simulink model "Auto_microgrid_forecasting_020822"  (R2020a)
settings: Solver=VariableStepAuto  StartTime=0.0  StopTime=50  MaxStep=1e-4  RelTol=1e-3
PreLoadFcn:
  | %run('FC_microgrid_param.m')
  | %load('gen_grid_init.mat')
InitFcn:
  | %load myisoModel_init;
  | run('FC_microgrid_param.m')
  | tic
  | run('CARTinitFcn.m')
  | %caseNo = 2;
  | 
  | %if (caseNo == 1)
  | %set_param(['Isolated_grid_paper_model_022521/SignalGen'], 'ActiveScenario', 'PStep222kW');
  | %else
  | %set_param(['Isolated_grid_paper_model_022521/SignalGen'], 'ActiveScenario', 'QStep222kVAr');
  | 
  | %end;
StopFcn:
  | toc
undefined symbols (not defined in the file or in its folder): breakpoints1, breakpoints2, cc_kp, cp_table_data, ctrl, D1, Delta, DiscIntNeverNeededParam, DT, FC_BESS, FC_PV_FirstSolar, find_system, Fnom, gcbh, libFC_BESS, libFC_PV, LowerLimit, magnitude, oversize, pll_ki, pll_kp, pq_ts, SOC_target, sps_rtmsupport, timer, Ts, ts, Ts_APC, Ts_Control, Ts_Power, UpperLimit
libraries: powerlib x151, simulink x100, powerlib_extras x100, powerlib_meascontrol x91, eePowerMeasurement x26, pi_ctrl x16, simulink_extras x12, sps_avr x7, eeGeneralControl x5, spsDieselMotorModel x3, libFSArray x2, SignalEditorBlockLib x2
(part 2 of 14)

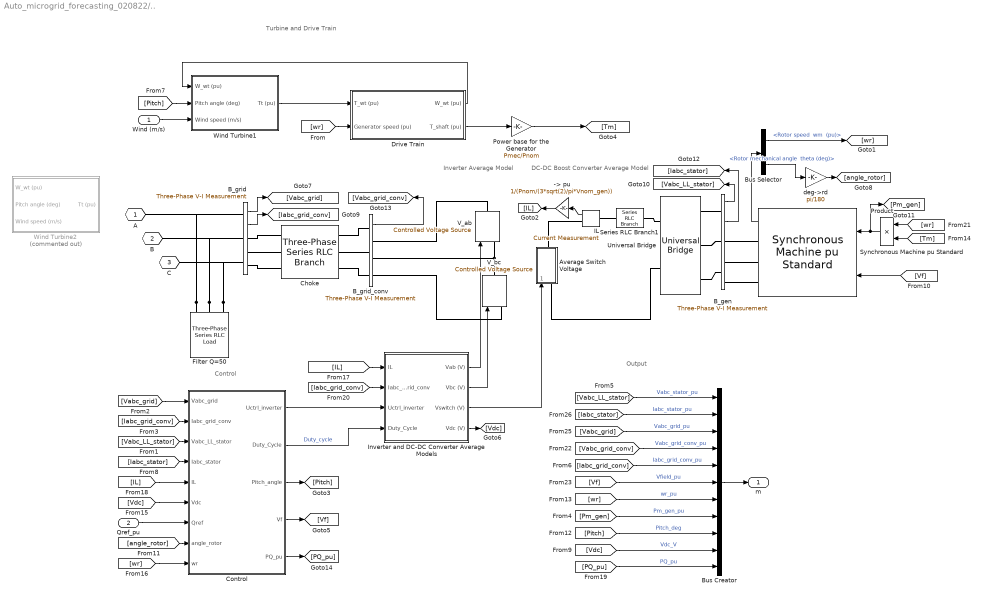
== system Auto_microgrid_forecasting_020822/.. ==
  note: DC-DC Boost Converter
      | Average Model
  note: Inverter
      | Average Model
  note: Output
  note: Control
  note: Turbine and Drive Train
  "Wind (m/s) " : Inport
  Qref_pu : Inport  Port=2
  -> pu : Gain  Gain=1/(Pnom/(3*sqrt(2)/pi*Vnom_gen))  SaturateOnIntegerOverflow=on  OutDataTypeStr=Inherit: Same as input  ParamDataTypeStr=Inherit: Same as input
  Average Switch Voltage : Subsystem
  B_gen : powerlib/Measurements/Three-Phase V-I Measurement  VoltageMeasurement=phase-to-phase  SetLabelV=off  LabelV=Vabc  Vpu=on  VpuLL=off  CurrentMeasurement=yes  SetLabelI=off  LabelI=Iabc  Ipu=on  Pbase=Pnom  Vbase=Vnom_gen  OutputType=Complex  PhasorSimulation=off  PSBequivalent=0
      settings: SourceProductBaseCode=MT,PS
  B_grid : powerlib/Measurements/Three-Phase V-I Measurement  VoltageMeasurement=phase-to-ground  SetLabelV=off  LabelV=Vabc  Vpu=on  VpuLL=off  CurrentMeasurement=yes  SetLabelI=off  LabelI=Iabc  Ipu=on  Pbase=Pnom  Vbase=Vnom  OutputType=Complex  PhasorSimulation=off  PSBequivalent=0
      settings: SourceProductBaseCode=MT,PS
  B_grid_conv : powerlib/Measurements/Three-Phase V-I Measurement  VoltageMeasurement=phase-to-ground  SetLabelV=off  LabelV=Vabc  Vpu=on  VpuLL=off  CurrentMeasurement=no  SetLabelI=off  LabelI=Iabc  Ipu=on  Pbase=Pnom  Vbase=Vnom  OutputType=Complex  PhasorSimulation=off  PSBequivalent=0
      settings: SourceProductBaseCode=MT,PS
  Bus Creator : BusCreator  Inputs=11
  Bus Selector : BusSelector  OutputSignals="Mechanical.Rotor speed  wm  (pu),Mechanical.Rotor mechanical angle  theta (deg)"
  "Choke " : powerlib/Elements/Three-Phase Series RLC Branch  LConnTagsString=A|B|C  RConnTagsString=A|B|C  BranchType=RL  Resistance=R_RL*Vnom^2/Pnom  Inductance=L_RL*Vnom^2/Pnom/(2*pi*Fnom)  Capacitance=[]  Measurements=None
      settings: SourceProductBaseCode=MT,PS
  Control : Subsystem
  Drive Train : Subsystem  mask(Wind Turbine shaft){H_WT=H_WT, Ksh=Ksh, D_mutual=D_mutual, wbase=2*pi*Fnom/p, w_wt0=w_wt0, torque0=torque0, Ts=Ts}
      mask prompts: H_WT "Wind turbine inertia constant H (s):"; Ksh "Shaft spring constant (pu of nominal mechanical torque/rad):"; D_mutual "Shaft mutual damping (pu of nominal mechanical torque/pu dw):"; wbase "Shaft base speed (rad/s):"; w_wt0 "Turbine initial speed (pu of base speed):"; torque0 "Initial output torque (pu of nominal mechanical torque):"; Ts "Sample time (s):"
      mask help:
      | This block implements a wind turbine drive train model. All shaft parameters are referred to high-speed shaft (generator shaft).
      |
      | The first input is the wind turbine torque in per unit (pu) based on the nominal power of the turbine and the base speed of the generator. The second input is the generator speed in pu based on the base speed of the generator.
      |
      | The outputs are:
      | 1- the transmitted torque of the shaft in pu based on the nominal power of the turbine and the base speed of the generator.
      | 2- the wind turbine speed in pu of the base speed of the generator.
  Filter Q=50 : powerlib/Elements/Three-Phase Series RLC Load  LConnTagsString=A|B|C  Configuration=Y (grounded)  NominalVoltage=Vnom  Vabc=[1e3 1e3 1e3]  Vabcp=[1e3 1e3 1e3]  NominalFrequency=Fnom  UnbalancedPower=off  ActivePower=C_var_filter/Q_filter  InductivePower=0  CapacitivePower=C_var_filter  Pabc=[10e3 9e3 11e3]  QLabc=[100 90 110]  QCabc=[100 90 110]  Pabcp=[10e3 9e3 11e3]  QLabcp=[100 90 110]  QCabcp=[100 90 110]  Measurements=None  LoadType=constant Z
      settings: SourceProductBaseCode=MT,PS
  IL : powerlib/Measurements/Current Measurement  PhasorSimulation=off  OutputType=Complex  PSBequivalent=0
      settings: SourceProductBaseCode=MT,PS
  Inverter and DC-DC Converter Average Models : Subsystem
  Power base for the Generator : Gain  Gain=Pmec/Pnom  SaturateOnIntegerOverflow=on  OutDataTypeStr=Inherit: Same as input  ParamDataTypeStr=Inherit: Same as input
  Product : Product  RndMeth=Zero
  Series RLC Branch1 : powerlib/Elements/Series RLC Branch  LConnTagsString=__new0  RConnTagsString=__new0  BranchType=RL  Resistance=R_Boost  Inductance=L_Boost  SetiL0=off  InitialCurrent=0  Capacitance=1.0  Setx0=off  InitialVoltage=0  Measurements=Branch current
      settings: SourceProductBaseCode=MT,PS
  Synchronous Machine pu Standard : powerlib/Machines/Synchronous Machine pu Standard  PresetModel=No  MechanicalLoad=Mechanical power Pm  ShowDetailedParameters=on  RotorType=Salient-pole  Units=per unit standard parameters  MeasurementBus=off  NominalParameters="[ Pnom  Vnom_gen Fnom ]"  Reactances1=[ 1.81, 0.3, 0.23, 1.76, 0.65, 0.25, 0.15 ]  Reactances2="[ Xd, Xd1, Xd2, Xq,  Xq2,  Xl ]"  dAxisTimeConstants=Open-circuit  qAxisTimeConstants=Short-circuit  TimeConstants1="[ 4.4849  0.0681  0.1  ]"  TimeConstants2=[ 8.0, 0.03, 1.0, 0.07 ]  TimeConstants3="[  Tdo1  Tdo2  Tq2  ]"  TimeConstants4=[ 8.0, 0.03, 0.3371, 0.0295 ]  TimeConstants5=[ 1.01, 0.053, 0.1 ]  TimeConstants6=[ 1.3201, 0.023, 1.0, 0.07 ]  TimeConstants7="[  1.01  0.053  0.051266  ]"  TimeConstants8=[ 1.3201, 0.0231, 0.3371, 0.0295 ]  StatorResistance=Resistance  Mechanical=[ H F p]  PolePairs=1  InitialConditions=init  SetSaturation=off  Saturation=[0.6404,0.7127,0.8441,0.9214,0.9956,1.082,1.19,1.316,1.457;0.7,0.7698,0.8872,0.9466,0.9969,1.046,1.1,1.151,1.201]  LoadFlowParameters=[1,0,0,0,0]  TsPowergui=0  TsBlock=-1  IterativeModel=Trapezoidal non iterative  IterativeDiscreteModel=Trapezoidal non iterative  BusType=PV  Pref=0  Qref=0  Qmin=-inf  Qmax=inf  PLF=0  QLF=0
      settings: SourceProductBaseCode=MT,PS
  Universal Bridge : powerlib/Power Electronics/Universal Bridge  Arms=3  SnubberResistance=2*Ts_snub/(Pnom/(1000*2*pi*Fnom*Vnom_gen^2))  SnubberCapacitance=Pnom/(1000*2*pi*Fnom*Vnom_gen^2)  Device=Diodes  Ron=1e-6/Nb_wt  Lon=0  ForwardVoltages="[  0  0  ]"  ForwardVoltage=0  GTOparameters=[ 10e-6 , 20e-6 ]  IGBTparameters=[ 1e-6 , 2e-6 ]  Measurements=None  Measurements_2=None  converterType=Rectifier
      settings: SourceProductBaseCode=MT,PS
  V_ab : powerlib/Electrical Sources/Controlled Voltage Source  Initialize=on  Source_Type=AC  Amplitude=0  Phase=0  Frequency=0  Measurements=None
      settings: SourceProductBaseCode=MT,PS
  V_bc : powerlib/Electrical Sources/Controlled Voltage Source  Initialize=on  Source_Type=AC  Amplitude=0  Phase=0  Frequency=0  Measurements=None
      settings: SourceProductBaseCode=MT,PS
  Wind Turbine1 : Subsystem  mask(Wind Turbine){Prated=Pmec, c1_c8=c1_c8, K1_K2=K1_K2, wind0=wind0, Ts=Ts}
      mask prompts: Prated "Nominal mechanical output power (W):"; c1_c8 "Coefficients [c1 ... c8]"; K1_K2 "Parameters [K1 K2]"; wind0 "Initial wind speed (m/s):"; Ts "Sample time (s):"
      mask help:
      | This block implements a generic wind turbine models.
      |
      | The first input is the turbine speed in per unit of the generator base speed. For a synchronous or asynchronous generator, the base speed is the synchronous speed. For a permanent-magnet generator, the base speed is defined as the speed producing nominal voltage at  no load. The second input is the blade pitch angle in degrees. The third input is the wind speed in m/s.
      |
      | The output is the torque applied to the drive train in per unit based on the nominal power of the turbine and the base speed of the generator.
      mask init:
      | c1 = c1_c8(1);
      | c2 = c1_c8(2);
      | c3 = c1_c8(3);
      | c4 = c1_c8(4);
      | c5 = c1_c8(5);
      | c6 = c1_c8(6);
      | c7 = c1_c8(7);;
      | c8 = c1_c8(8);
      | 
      | K1=K1_K2(1);
      | K2=K1_K2(2);
      settings: OpenFcn=power_openblockproxy();
      mask Display: disp('');
  Wind Turbine2 : Subsystem  Commented=on  mask(Wind Turbine){Prated=Pmec, c1_c8=c1_c8, K1_K2=K1_K2, wind0=wind0, Ts=Ts}
      mask prompts: Prated "Nominal mechanical output power (W):"; c1_c8 "Coefficients [c1 ... c8]"; K1_K2 "Parameters [K1 K2]"; wind0 "Initial wind speed (m/s):"; Ts "Sample time (s):"
      mask help:
      | This block implements a generic wind turbine models.
      |
      | The first input is the turbine speed in per unit of the generator base speed. For a synchronous or asynchronous generator, the base speed is the synchronous speed. For a permanent-magnet generator, the base speed is defined as the speed producing nominal voltage at  no load. The second input is the blade pitch angle in degrees. The third input is the wind speed in m/s.
      |
      | The output is the torque applied to the drive train in per unit based on the nominal power of the turbine and the base speed of the generator.
      mask init:
      | c1 = c1_c8(1);
      | c2 = c1_c8(2);
      | c3 = c1_c8(3);
      | c4 = c1_c8(4);
      | c5 = c1_c8(5);
      | c6 = c1_c8(6);
      | c7 = c1_c8(7);;
      | c8 = c1_c8(8);
      | 
      | K1=K1_K2(1);
      | K2=K1_K2(2);
      settings: OpenFcn=power_openblockproxy();
      mask Display: disp('');
  deg->rd : Gain  Gain=pi/180  SaturateOnIntegerOverflow=on  OutDataTypeStr=Inherit: Same as input  ParamDataTypeStr=Inherit: Same as input
  A : PMIOPort  Tag=PMCPort  Side=Left
  B : PMIOPort  Tag=PMCPort  Port=2  Side=Left
  C : PMIOPort  Tag=PMCPort  Port=3  Side=Left
  m : Outport  VectorParamsAs1DForOutWhenUnconnected=off
  wires:
  -> pu/1 -> [IL]
  [IL] -> Control/5(IL)
  [PQ_pu] -> Bus Creator/11  "PQ_pu"
  Control/5(PQ_pu) -> [PQ_pu]
  Inverter and DC-DC Converter Average Models/2(Vbc (V)) -> V_bc/1
  Inverter and DC-DC Converter Average Models/1(Vab (V)) -> V_ab/1
  [Vf] -> Synchronous Machine pu Standard/2
  Inverter and DC-DC Converter Average Models/4(Vdc (V)) -> [Vdc]
  Control/4(Vf) -> [Vf]
  Control/3(Pitch_angle) -> [Pitch]
  Control/2(Duty_Cycle) -> Inverter and DC-DC Converter Average Models/4(Duty_Cycle)  "Duty_cycle"
  Control/1(Uctrl_inverter) -> Inverter and DC-DC Converter Average Models/3(Uctrl_inverter)
  [wr] -> Control/9(wr)
  [angle_rotor] -> Control/8(angle_rotor)
  Qref_pu/1 -> Control/7(Qref)
  [Vdc] -> Control/6(Vdc)
  [Iabc_stator] -> Control/4(Iabc_stator)
  [Vabc_LL_stator] -> Control/3(Vabc_LL_stator)
  [Iabc_grid_conv] -> Control/2(Iabc_grid_conv)
  [Vabc_grid] -> Control/1(Vabc_grid)
  B_gen/2 -> [Iabc_stator]
  B_gen/1 -> [Vabc_LL_stator]
  B_grid/2 -> [Iabc_grid_conv]
  B_grid/1 -> [Vabc_grid]
  [IL] -> Inverter and DC-DC Converter Average Models/1(IL)
  IL/1 -> -> pu/1
  Inverter and DC-DC Converter Average Models/3(Vswitch (V)) -> Average Switch Voltage/1(Vswitch)
  [Iabc_grid_conv] -> Inverter and DC-DC Converter Average Models/2(Iabc_grid_conv)
  Product/1 -> [Pm_gen], Synchronous Machine pu Standard/1
  [Tm] -> Product/2
  [Vdc] -> Bus Creator/10  "Vdc_V"
  [Pitch] -> Bus Creator/9  "Pitch_deg"
  [Pm_gen] -> Bus Creator/8  "Pm_gen_pu"
  [wr] -> Bus Creator/7  "wr_pu"
  [Vf] -> Bus Creator/6  "Vfield_pu"
  [Iabc_grid_conv] -> Bus Creator/5  "Iabc_grid_conv_pu"
  [Vabc_grid_conv] -> Bus Creator/4  "Vabc_grid_conv_pu"
  Bus Creator/1 -> m/1
  [Vabc_grid] -> Bus Creator/3  "Vabc_grid_pu"
  [Iabc_stator] -> Bus Creator/2  "Iabc_stator_pu"
  [Vabc_LL_stator] -> Bus Creator/1  "Vabc_stator_pu"
  B_grid_conv/1 -> [Vabc_grid_conv]
  Synchronous Machine pu Standard/1 -> Bus Selector/1
  [wr] -> Product/1
  Bus Selector/1 -> [wr]  "<Rotor speed  wm  (pu)>"
  deg->rd/1 -> [angle_rotor]
  Bus Selector/2 -> deg->rd/1  "<Rotor mechanical angle  theta (deg)>"
  [Pitch] -> Wind Turbine1/2(Pitch angle (deg))
  Drive Train/1(W_wt (pu)) -> Wind Turbine1/1(W_wt (pu))
  "Wind (m/s) "/1 -> Wind Turbine1/3(Wind speed (m/s))
  Power base for the Generator/1 -> [Tm]
  Drive Train/2(T_shaft (pu)) -> Power base for the Generator/1
  [wr] -> Drive Train/2(Generator speed (pu))
  Wind Turbine1/1(Tt (pu)) -> Drive Train/1(T_wt (pu))
  connections:
  Average Switch Voltage/RConn1 -- IL/RConn1
  Series RLC Branch1/RConn1 -- IL/LConn1
  Universal Bridge/LConn3 -- B_gen/LConn3
  Universal Bridge/LConn2 -- B_gen/LConn2
  Universal Bridge/LConn1 -- B_gen/LConn1
  B_grid_conv/RConn2 -- V_ab/LConn1 -- V_bc/RConn1
  B_grid_conv/RConn3 -- V_bc/LConn1
  V_ab/RConn1 -- B_grid_conv/RConn1
  Average Switch Voltage/LConn1 -- Universal Bridge/RConn2
  Series RLC Branch1/LConn1 -- Universal Bridge/RConn1
  "Choke "/RConn3 -- B_grid_conv/LConn3
  "Choke "/RConn2 -- B_grid_conv/LConn2
  "Choke "/RConn1 -- B_grid_conv/LConn1
  Filter Q=50/LConn3 -- B_grid/LConn3 -- C/RConn1
  Filter Q=50/LConn2 -- B_grid/LConn2 -- B/RConn1
  Filter Q=50/LConn1 -- A/RConn1 -- B_grid/LConn1
  B_grid/RConn3 -- "Choke "/LConn3
  B_grid/RConn2 -- "Choke "/LConn2
  B_grid/RConn1 -- "Choke "/LConn1
  B_gen/RConn3 -- Synchronous Machine pu Standard/RConn3
  B_gen/RConn2 -- Synchronous Machine pu Standard/RConn2
  B_gen/RConn1 -- Synchronous Machine pu Standard/RConn1

== system Auto_microgrid_forecasting_020822/Control1 ==
  Bus Creator : BusCreator  Inputs=6
  Bus Selector : BusSelector  OutputSignals=PV PQ cmd,f setpoint,V setpoint,PV switch,PV_mode
  Constant2 : Constant  Commented=on
  Constant3 : Constant  Commented=on
  Demux1 : Demux  Outputs=2
  Step2 : Step  Before=1  After=0
  Out1 : Outport
  wires:
  Bus Selector/3 -> Bus Creator/4  "<V setpoint>"
  Bus Creator/1 -> Out1/1
  Bus Selector/2 -> Bus Creator/3  "<f setpoint>"
  Bus Selector/5 -> Bus Creator/5  "<PV_mode>"
  Demux1/2 -> Bus Creator/2  "q_ref"
  Demux1/1 -> Bus Creator/1  "p_ref"
  Bus Selector/4 -> Bus Creator/6  "<PV switch>"
  [MGCC_cmd] -> Bus Selector/1
  Bus Selector/1 -> Demux1/1  "<PV PQ cmd>"
  Constant3/1 -> ?  "V setpoint"
  Constant2/1 -> ?  "f setpoint"

== system Auto_microgrid_forecasting_020822/Control3 ==
  Bus Creator : BusCreator  Inputs=5
  Constant1 : Constant  SampleTime=-1
  Constant2 : Constant  SampleTime=-1
  Constant3 : Constant  Value=-1  SampleTime=-1
  Constant5 : Constant  Value=0  SampleTime=-1
  Step1 : Step  Time=1000
  Control : Outport
  wires:
  Constant3/1 -> Bus Creator/1  "p_ref"
  Constant5/1 -> Bus Creator/2  "q_ref"
  Step1/1 -> Bus Creator/5  "GF_mode"
  Constant1/1 -> Bus Creator/3  "f_ref"
  Bus Creator/1 -> Control/1
  Constant2/1 -> Bus Creator/4  "v_ref"

== system Auto_microgrid_forecasting_020822/Defferable Load (0-446.25 kW) ==
  Control : Inport
  Demux : Demux  Outputs=8
      settings: DisplayOption=none
  Resistive Loads : Subsystem
  Switches : Subsystem
  A : PMIOPort  Side=Left
  B : PMIOPort  Port=2  Side=Left
  C : PMIOPort  Port=3  Side=Left
  wires:
  Control/1 -> Demux/1
  Demux/8 -> Switches/8(P_ABC7)
  Demux/7 -> Switches/7(P_ABC6)
  Demux/6 -> Switches/6(P_ABC5)
  Demux/5 -> Switches/5(P_ABC4)
  Demux/4 -> Switches/4(P_ABC3)
  Demux/3 -> Switches/3(P_ABC2)
  Demux/2 -> Switches/2(P_ABC1)
  Demux/1 -> Switches/1(P_ABC0)
  connections:
  Switches/RConn1 -- Resistive Loads/LConn1
  Switches/RConn2 -- Resistive Loads/LConn2
  Switches/RConn3 -- Resistive Loads/LConn3
  Switches/RConn4 -- Resistive Loads/LConn4
  Switches/RConn5 -- Resistive Loads/LConn5
  Switches/RConn6 -- Resistive Loads/LConn6
  Switches/RConn7 -- Resistive Loads/LConn7
  Switches/RConn8 -- Resistive Loads/LConn8
  Switches/RConn9 -- Resistive Loads/LConn9
  Switches/RConn10 -- Resistive Loads/LConn10
  Switches/RConn11 -- Resistive Loads/LConn11
  Switches/RConn12 -- Resistive Loads/LConn12
  Switches/RConn13 -- Resistive Loads/LConn13
  Switches/RConn14 -- Resistive Loads/LConn14
  Switches/RConn15 -- Resistive Loads/LConn15
  Switches/RConn16 -- Resistive Loads/LConn16
  Switches/RConn17 -- Resistive Loads/LConn17
  Switches/RConn18 -- Resistive Loads/LConn18
  Switches/RConn19 -- Resistive Loads/LConn19
  Switches/RConn20 -- Resistive Loads/LConn20
  Switches/RConn21 -- Resistive Loads/LConn21
  Switches/RConn22 -- Resistive Loads/LConn22
  Switches/RConn23 -- Resistive Loads/LConn23
  Switches/RConn24 -- Resistive Loads/LConn24
  A/RConn1 -- Switches/LConn1
  B/RConn1 -- Switches/LConn2
  C/RConn1 -- Switches/LConn3

== system Auto_microgrid_forecasting_020822/Discrete Frequency Regulator ==
  Vabc : Inport
  +/- 0.005 Hz : DeadZone  LowerValue=-0.005  UpperValue=0.005  SaturateOnIntegerOverflow=on
  Discrete PID Controller : Subsystem  DialogController=POWERSYS.PowerSysDialog  mask(Discrete PID Controller){Kp=Kp, Ki=0, Kd=Kd, TcD=0.5e-3, Par_Limits=[255 0], Init=0, Ts=Ts}
      mask prompts: Kp "Proportional gain (Kp):"; Ki "Integral gain (Ki):"; Kd "Derivative gain (Kd):"; TcD "Time constant for derivative (s):"; Par_Limits "Output limits: [ Upper   Lower ]"; Init "Output initial value:"; Ts "Sample time:"
      mask help: This block implements a discrete PID controller.
      mask init:
      | UpperLimit=Par_Limits(1);
      | LowerLimit=Par_Limits(2);
      | power_initmask();
      mask Help: This block is part of a subset of blocks in the Extras library that does not have documentation associated with it, other than the block mask description.
      mask Display: disp('PID');
  Discrete-Time Integrator : DiscreteIntegrator  SampleTime=Ts  LimitOutput=on  UpperSaturationLimit=1  LowerSaturationLimit=0  ICPrevOutput=DiscIntNeverNeededParam  ICPrevScaledInput=DiscIntNeverNeededParam
  PLL (3ph) : powerlib_meascontrol/PLL/PLL (3ph)  Fmin=45  Par_Init=[0 Freq_ref]  ParK=[60 1400]  TcD=2e-4  MaxRateChangeFreq=12  FilterCutOffFreq=25  Ts=Ts  AGC=on
      settings: SourceProductBaseCode=MT,PS
  Pulses Decoder : Subsystem  mask(Pulses Decoder){n=8}
      mask prompts: n "Number of bits to decode:"
      mask help:
      | Decode the scalar input 'Code' into a vector output 'Pulses' based on  the specified number of bits to decode.
      | (Element 1 of vector output = least significant bit)
  Reference Frequency : Constant  Value=Freq_ref
  Sampling system : Subsystem
  Sum : Sum  Inputs=|+-  InputSameDT=on  SaturateOnIntegerOverflow=on  OutDataTypeStr=Inherit: Same as first input
  Terminator : Terminator
  Control : Outport  VectorParamsAs1DForOutWhenUnconnected=off
  tag scope: Freq=global
  wires:
  Vabc/1 -> PLL (3ph)/1
  PLL (3ph)/2 -> Terminator/1
  Sampling system/1(Pulses_ABC0_7) -> Control/1
  Discrete-Time Integrator/1 -> Discrete PID Controller/1(Error)
  Reference Frequency/1 -> Sum/2
  Discrete PID Controller/1(Out) -> Pulses Decoder/1(Code)
  Sum/1 -> +/- 0.005 Hz/1
  Pulses Decoder/1(Pulses) -> Sampling system/1(BITA0_7)
  +/- 0.005 Hz/1 -> Discrete-Time Integrator/1
  PLL (3ph)/1 -> Sum/1, [Freq]

== system Auto_microgrid_forecasting_020822/FC_BESS ==
  Control : Inport
  Battery : Subsystem  BlockChoice=LG_Battery
      link override LG_Battery/LG 1-MW//1-MWh BESS: NomQ=1e3/100  SOC=20
      settings: AttributesFormatString=%<BlockChoice>  MemberBlocks=LG_Battery,NoBattery
      settings: TemplateBlock=|
      | libLgBattery/Configurable
      | Subsystem
  SMAInverter : Subsystem
  Scope : Scope  Commented=on  NumInputPorts=2
  Transformer 1-MVA 13.2-kV/400-V : powerlib/Elements/Three-Phase Transformer (Two Windings)  Winding1Connection=Delta (D1)  Winding2Connection=Yg  CoreType=Three single-phase transformers  SetSaturation=off  Hysteresis=off  DataFile='hysteresis'  SetInitialFlux=off  Measurements=None  UNITS=pu  NominalPower=[ 1e6 , 60 ]  Winding1=[13.2e+3 0.003 0.03]  Winding2=[400 0.003 0.03]  Rm=500.02  Lm=500  L0=0.5  Saturation=[0 0;0.0024 1.2;1 1.52]  InitialFluxes=[ 0.8 , -0.8 , 0.7 ]  BreakLoop=off  DiscreteSolver=Trapezoidal iterative  DataType=off  TransfoNumber=1
  A : PMIOPort  Side=Left
  B : PMIOPort  Port=2  Side=Left
  C : PMIOPort  Port=3  Side=Left
  m : Outport
  wires:
  Battery/2(m) -> m/1
  Battery/1(Vdc) -> Scope/1, SMAInverter/1(Vdc)
  SMAInverter/1(Idc) -> Scope/2, Battery/1(Idc)
  Control/1 -> SMAInverter/2(Control)
  connections:
  Transformer 1-MVA 13.2-kV/400-V/LConn1 -- A/RConn1
  Transformer 1-MVA 13.2-kV/400-V/LConn2 -- B/RConn1
  Transformer 1-MVA 13.2-kV/400-V/RConn1 -- SMAInverter/LConn1
  Transformer 1-MVA 13.2-kV/400-V/LConn3 -- C/RConn1
  Transformer 1-MVA 13.2-kV/400-V/RConn3 -- SMAInverter/LConn3
  Transformer 1-MVA 13.2-kV/400-V/RConn2 -- SMAInverter/LConn2

== system Auto_microgrid_forecasting_020822/FC_PV_FirstSolar ==
  Control : Inport
  Irradiance : Inport  Port=2
  AllStringInverters : Subsystem
  Bus Selector : BusSelector  OutputSignals=V_PV,I_PV
  Gain : Gain  Gain=-1
  Gain1 : Gain  Gain=-1
  MPPT Parameters : Subsystem  mask(MPPT Parameters){Increment_MPPT=0.01, Limits_MPPT=[1450 600], Vdc_ref_Init=600}
      mask prompts: Increment_MPPT "Output increment(V)"; Limits_MPPT "Output limits [Upper Lower]"; Vdc_ref_Init "Output initial value (V)"
      mask help:
      | MPPT Controller using Perturbe & Observe technique
      |
      | Initial value for Vdc_ref output (Dinit)
      | Upper limit for Vdc_ref (Dmax)
      | Lower limit for Vdc_ref (Dmax)
      | Increment value used to increase/decrease Vdc_ref (DeltaD)
  "MPPT Controller using Perturbe & Observe technique " : MATLAB Function  TreatAsAtomicUnit=on
  MPPT Enable : Constant  Value=0
  PV_Array : Subsystem  BlockChoice=FS_Array
      settings: AttributesFormatString=%<BlockChoice>  MemberBlocks=FS_Array,No_Array
      settings: TemplateBlock=|
      | libFSArray/Configurable
      | Subsystem
  Switch : Switch  Criteria=u2 ~= 0
  Transformer  750kW 13.2-kV/600-V : powerlib/Elements/Three-Phase Transformer (Two Windings)  Winding1Connection=Delta (D1)  Winding2Connection=Yg  CoreType=Three single-phase transformers  SetSaturation=off  Hysteresis=off  DataFile='hysteresis'  SetInitialFlux=off  Measurements=None  UNITS=pu  NominalPower=[ 0.5e6 , 60 ]  Winding1=[13.2e+3 0.003 0.03]  Winding2=[600 0.003 0.03]  Rm=500.02  Lm=inf  L0=0.5  Saturation=[0 0;0.0024 1.2;1 1.52]  InitialFluxes=[ 0.8 , -0.8 , 0.7 ]  BreakLoop=off  DiscreteSolver=Trapezoidal iterative  DataType=off  TransfoNumber=1
  A : PMIOPort  Side=Left
  B : PMIOPort  Port=2  Side=Left
  C : PMIOPort  Port=3  Side=Left
  m : Outport
  wires:
  Control/1 -> AllStringInverters/2(Control)
  PV_Array/1(Idc) -> Gain/1
  Irradiance/1 -> PV_Array/2(Irradiance)
  PV_Array/2(m) -> Bus Selector/1, m/1
  MPPT Enable/1 -> "MPPT Controller using Perturbe & Observe technique "/2(Enabled), Switch/2
  AllStringInverters/1(Udc) -> Gain1/1
  MPPT Parameters/1(Param) -> "MPPT Controller using Perturbe & Observe technique "/1(Param)
  Bus Selector/1 -> [V_PV]  "<V_PV>"
  Bus Selector/2 -> [I_PV]  "<I_PV>"
  [V_PV] -> "MPPT Controller using Perturbe & Observe technique "/3(V)
  [I_PV] -> "MPPT Controller using Perturbe & Observe technique "/4(I)
  Switch/1 -> PV_Array/1(Vdc)
  "MPPT Controller using Perturbe & Observe technique "/1(D) -> Switch/3
  Gain/1 -> AllStringInverters/1(Idc)
  Gain1/1 -> Switch/1
  connections:
  Transformer  750kW 13.2-kV/600-V/RConn2 -- AllStringInverters/LConn2
  Transformer  750kW 13.2-kV/600-V/RConn3 -- AllStringInverters/LConn3
  Transformer  750kW 13.2-kV/600-V/LConn3 -- C/RConn1
  Transformer  750kW 13.2-kV/600-V/RConn1 -- AllStringInverters/LConn1
  Transformer  750kW 13.2-kV/600-V/LConn2 -- B/RConn1
  Transformer  750kW 13.2-kV/600-V/LConn1 -- A/RConn1

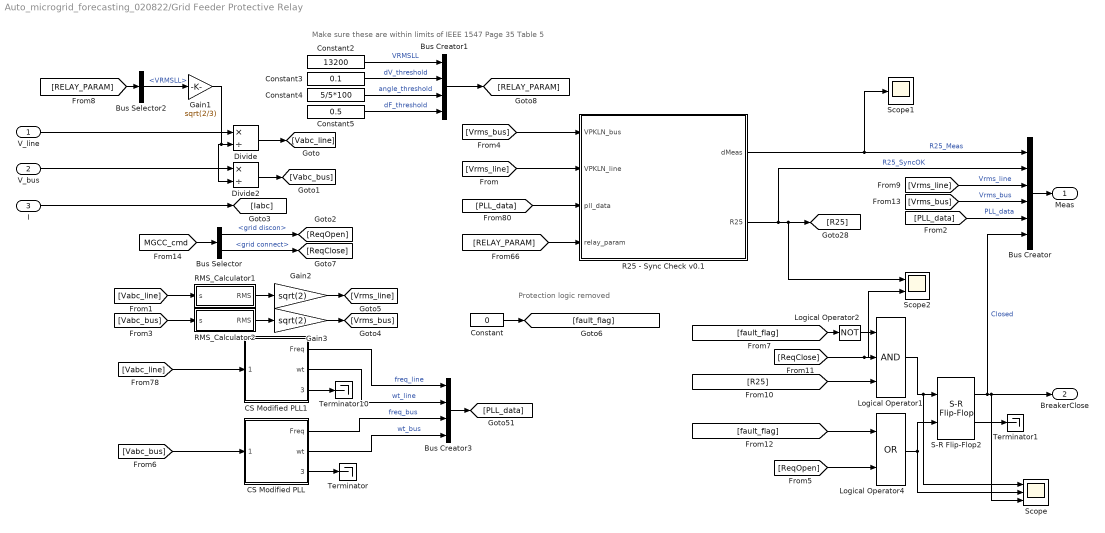
== system Auto_microgrid_forecasting_020822/Grid Feeder Protective Relay ==
  note: Make sure these are within limits of IEEE 1547 Page 35 Table 5
  note: Protection logic removed
  V_line : Inport
  V_bus : Inport  Port=2
  I : Inport  Port=3
  Bus Creator : BusCreator  Inputs=6
  Bus Creator1 : BusCreator  Inputs=4
  Bus Creator3 : BusCreator  Inputs=4
  Bus Selector : BusSelector  OutputSignals=grid discon,grid connect
  Bus Selector2 : BusSelector  OutputSignals=VRMSLL
  CS Modified PLL : Subsystem  DialogController=POWERSYS.PowerSysDialog  mask(Discrete 3-phase PLL){Flim=[55 66], Par_Init=[0 60], ParK=[ 180 3200 1 ], Ts=Ts, AGC=off}
      mask prompts: Flim "Frequency limits (Hz):"; Par_Init "Initial inputs:[ Phase(degrees)   Frequency(Hz) ]"; ParK "Regulator gains [ Kp  Ki  Kd ]"; Ts "Sample time:"; AGC "Enable Automatic Gain Control"
      mask help:
      | This Phase Locked Loop (PLL) system can be used  to synchronize on a set of variable frequency, three-phase sinusoidal signals. If the Automatic Gain Control is enabled, the input (phase error) of the PLL regulator is scaled according to the input signals magnitude.
      |
      | For optimal performance, the following settings are recommended:
      |   [ Kp Ki  Kd ] = [ 180  3200  1 ]
      |   "Enable Automatic Gain Control" checked
      |
      | Input 1: Vector containing the normalized three-phase signals [Va Vb Vc]
      | Output 1:  Measured frequency (Hz) = w/(2pi)
      | Output 2:  Ramp w.t varying between  0 and 2*pi,
      |      synchronized on zero crossings of the fundamental (positive-sequence) of phase A.
      | Output 3: Vector [sin(wt) cos(wt)]
      mask init:
      | Kp=ParK(1);
      | Ki=ParK(2);
      | if length(ParK)==2
      |     Kd=0;
      | else
      |     Kd=ParK(3);
      | end    
      | Phase_Init=Par_Init(1);
      | Finit=Par_Init(2);
      | %power_initmask();
      settings: OpenFcn=power_openblockproxy();
      mask Display: disp('')
  CS Modified PLL1 : Subsystem  DialogController=POWERSYS.PowerSysDialog  mask(Discrete 3-phase PLL){Flim=[55 66], Par_Init=[0 60], ParK=[ 180 3200 1 ], Ts=Ts, AGC=off}
      mask prompts: Flim "Frequency limits (Hz):"; Par_Init "Initial inputs:[ Phase(degrees)   Frequency(Hz) ]"; ParK "Regulator gains [ Kp  Ki  Kd ]"; Ts "Sample time:"; AGC "Enable Automatic Gain Control"
      mask help:
      | This Phase Locked Loop (PLL) system can be used  to synchronize on a set of variable frequency, three-phase sinusoidal signals. If the Automatic Gain Control is enabled, the input (phase error) of the PLL regulator is scaled according to the input signals magnitude.
      |
      | For optimal performance, the following settings are recommended:
      |   [ Kp Ki  Kd ] = [ 180  3200  1 ]
      |   "Enable Automatic Gain Control" checked
      |
      | Input 1: Vector containing the normalized three-phase signals [Va Vb Vc]
      | Output 1:  Measured frequency (Hz) = w/(2pi)
      | Output 2:  Ramp w.t varying between  0 and 2*pi,
      |      synchronized on zero crossings of the fundamental (positive-sequence) of phase A.
      | Output 3: Vector [sin(wt) cos(wt)]
      mask init:
      | Kp=ParK(1);
      | Ki=ParK(2);
      | if length(ParK)==2
      |     Kd=0;
      | else
      |     Kd=ParK(3);
      | end    
      | Phase_Init=Par_Init(1);
      | Finit=Par_Init(2);
      | %power_initmask();
      settings: OpenFcn=power_openblockproxy();
      mask Display: disp('')
  Constant : Constant  Value=0
  Constant2 : Constant  Value=13200
  Constant3 : Constant  Value=0.1
  Constant4 : Constant  Value=5/5*100
  Constant5 : Constant  Value=0.5
  Divide : Product  Inputs=*/
  Divide2 : Product  Inputs=*/
  Gain1 : Gain  Gain=sqrt(2/3)
  Gain2 : Gain  Gain=sqrt(2)
  Gain3 : Gain  Gain=sqrt(2)
  Logical Operator1 : Logic  Inputs=3  AllPortsSameDT=off  OutDataTypeStr=boolean
  Logical Operator2 : Logic  Operator=NOT  AllPortsSameDT=off  OutDataTypeStr=boolean
  Logical Operator4 : Logic  Operator=OR  AllPortsSameDT=off  OutDataTypeStr=boolean
  R25 - Sync Check v0.1 : Subsystem  mask(Relay synch check){Ts=Ts}
      mask prompts: Ts "Sampling Time [Sec]"
      mask help:
      | This block checks if the the specified conditions for breaker reclosing
      | are met at both terminals of the circuit breaker. This synch check is
      | intended for use in bus-ties, and service lines.
      |
      | The input bus with the relay parameters should be ordered as follows:
      | 1) VRMSLL
      | 2) IOC
      | 3) TOC
      | 4) dV_threshold
      | 5) angle_threshold
      | 6) dF_threshold
  RMS_Calculator1 : Subsystem  mask{Ts=Ts}
      mask prompts: Ts "Sample Time [Sec]"
  RMS_Calculator2 : Subsystem  mask{Ts=Ts}
      mask prompts: Ts "Sample Time [Sec]"
  S-R Flip-Flop2 : simulink_extras/Flip Flops/S-R Flip-Flop  initial_condition=1
  Scope : Scope  NumInputPorts=3
  Scope1 : Scope
  Scope2 : Scope  NumInputPorts=2
  Terminator : Terminator
  Terminator1 : Terminator
  Terminator10 : Terminator
  Meas : Outport
  BreakerClose : Outport  Port=2
  wires:
  V_line/1 -> Divide/1
  Bus Creator3/1 -> [PLL_data]
  CS Modified PLL1/3(Sin_Cos) -> Terminator10/1
  CS Modified PLL1/1(Freq) -> Bus Creator3/1  "freq_line"
  CS Modified PLL/1(Freq) -> Bus Creator3/3  "freq_bus"
  CS Modified PLL/3(Sin_Cos) -> Terminator/1
  [Vabc_bus] -> CS Modified PLL/1(Vabc(pu))
  CS Modified PLL/2(wt) -> Bus Creator3/4  "wt_bus"
  CS Modified PLL1/2(wt) -> Bus Creator3/2  "wt_line"
  [Vabc_line] -> CS Modified PLL1/1(Vabc(pu))
  R25 - Sync Check v0.1/1(dMeas) -> Scope1/1, Bus Creator/1  "R25_Meas"
  [PLL_data] -> R25 - Sync Check v0.1/3(pll_data)
  [Vrms_line] -> R25 - Sync Check v0.1/2(VPKLN_line)
  [Vrms_bus] -> R25 - Sync Check v0.1/1(VPKLN_bus)
  [RELAY_PARAM] -> R25 - Sync Check v0.1/4(relay_param)
  R25 - Sync Check v0.1/2(R25) -> Bus Creator/2, Scope2/1, [R25]  "R25_SyncOK"
  V_bus/1 -> Divide2/1
  I/1 -> [Iabc]
  [Vabc_line] -> RMS_Calculator1/1(s)
  [Vabc_bus] -> RMS_Calculator2/1(s)
  RMS_Calculator2/1(RMS) -> Gain3/1
  RMS_Calculator1/1(RMS) -> Gain2/1
  [ReqClose] -> Scope2/2, Logical Operator1/2
  Logical Operator4/1 -> S-R Flip-Flop2/2, Scope/2
  [fault_flag] -> Logical Operator2/1
  S-R Flip-Flop2/1 -> BreakerClose/1, Scope/3, Bus Creator/6  "Closed"
  Logical Operator2/1 -> Logical Operator1/1
  [fault_flag] -> Logical Operator4/1
  Logical Operator1/1 -> Scope/1, S-R Flip-Flop2/1
  S-R Flip-Flop2/2 -> Terminator1/1
  [R25] -> Logical Operator1/3
  Constant/1 -> [fault_flag]
  Bus Selector/1 -> [ReqOpen]  "<grid discon>"
  Bus Selector/2 -> [ReqClose]  "<grid connect>"
  [ReqOpen] -> Logical Operator4/2
  Bus Creator/1 -> Meas/1
  Constant3/1 -> Bus Creator1/2  "dV_threshold"
  Constant2/1 -> Bus Creator1/1  "VRMSLL"
  Constant4/1 -> Bus Creator1/3  "angle_threshold"
  Constant5/1 -> Bus Creator1/4  "dF_threshold"
  Bus Creator1/1 -> [RELAY_PARAM]
  Gain1/1 -> Divide2/2, Divide/2
  [RELAY_PARAM] -> Bus Selector2/1
  Bus Selector2/1 -> Gain1/1  "<VRMSLL>"
  Divide/1 -> [Vabc_line]
  Divide2/1 -> [Vabc_bus]
  Gain2/1 -> [Vrms_line]
  Gain3/1 -> [Vrms_bus]
  [PLL_data] -> Bus Creator/5  "PLL_data"
  [Vrms_line] -> Bus Creator/3  "Vrms_line"
  [Vrms_bus] -> Bus Creator/4  "Vrms_bus"
  [MGCC_cmd] -> Bus Selector/1

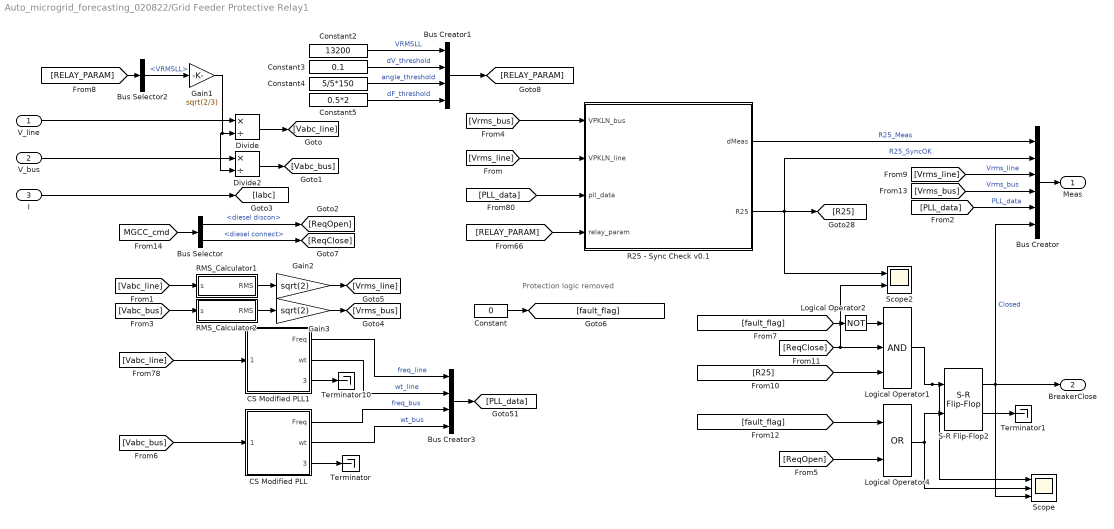
== system Auto_microgrid_forecasting_020822/Grid Feeder Protective Relay1 ==
  note: Protection logic removed
  V_line : Inport
  V_bus : Inport  Port=2
  I : Inport  Port=3
  Bus Creator : BusCreator  Inputs=6
  Bus Creator1 : BusCreator  Inputs=4
  Bus Creator3 : BusCreator  Inputs=4
  Bus Selector : BusSelector  OutputSignals=diesel discon,diesel connect
  Bus Selector2 : BusSelector  OutputSignals=VRMSLL
  CS Modified PLL : Subsystem  DialogController=POWERSYS.PowerSysDialog  mask(Discrete 3-phase PLL){Flim=[55 66], Par_Init=[0 60], ParK=[ 180 3200 1 ], Ts=Ts, AGC=off}
      mask prompts: Flim "Frequency limits (Hz):"; Par_Init "Initial inputs:[ Phase(degrees)   Frequency(Hz) ]"; ParK "Regulator gains [ Kp  Ki  Kd ]"; Ts "Sample time:"; AGC "Enable Automatic Gain Control"
      mask help:
      | This Phase Locked Loop (PLL) system can be used  to synchronize on a set of variable frequency, three-phase sinusoidal signals. If the Automatic Gain Control is enabled, the input (phase error) of the PLL regulator is scaled according to the input signals magnitude.
      |
      | For optimal performance, the following settings are recommended:
      |   [ Kp Ki  Kd ] = [ 180  3200  1 ]
      |   "Enable Automatic Gain Control" checked
      |
      | Input 1: Vector containing the normalized three-phase signals [Va Vb Vc]
      | Output 1:  Measured frequency (Hz) = w/(2pi)
      | Output 2:  Ramp w.t varying between  0 and 2*pi,
      |      synchronized on zero crossings of the fundamental (positive-sequence) of phase A.
      | Output 3: Vector [sin(wt) cos(wt)]
      mask init:
      | Kp=ParK(1);
      | Ki=ParK(2);
      | if length(ParK)==2
      |     Kd=0;
      | else
      |     Kd=ParK(3);
      | end    
      | Phase_Init=Par_Init(1);
      | Finit=Par_Init(2);
      | %power_initmask();
      settings: OpenFcn=power_openblockproxy();
      mask Display: disp('')
  CS Modified PLL1 : Subsystem  DialogController=POWERSYS.PowerSysDialog  mask(Discrete 3-phase PLL){Flim=[55 66], Par_Init=[0 60], ParK=[ 180 3200 1 ], Ts=Ts, AGC=off}
      mask prompts: Flim "Frequency limits (Hz):"; Par_Init "Initial inputs:[ Phase(degrees)   Frequency(Hz) ]"; ParK "Regulator gains [ Kp  Ki  Kd ]"; Ts "Sample time:"; AGC "Enable Automatic Gain Control"
      mask help:
      | This Phase Locked Loop (PLL) system can be used  to synchronize on a set of variable frequency, three-phase sinusoidal signals. If the Automatic Gain Control is enabled, the input (phase error) of the PLL regulator is scaled according to the input signals magnitude.
      |
      | For optimal performance, the following settings are recommended:
      |   [ Kp Ki  Kd ] = [ 180  3200  1 ]
      |   "Enable Automatic Gain Control" checked
      |
      | Input 1: Vector containing the normalized three-phase signals [Va Vb Vc]
      | Output 1:  Measured frequency (Hz) = w/(2pi)
      | Output 2:  Ramp w.t varying between  0 and 2*pi,
      |      synchronized on zero crossings of the fundamental (positive-sequence) of phase A.
      | Output 3: Vector [sin(wt) cos(wt)]
      mask init:
      | Kp=ParK(1);
      | Ki=ParK(2);
      | if length(ParK)==2
      |     Kd=0;
      | else
      |     Kd=ParK(3);
      | end    
      | Phase_Init=Par_Init(1);
      | Finit=Par_Init(2);
      | %power_initmask();
      settings: OpenFcn=power_openblockproxy();
      mask Display: disp('')
  Constant : Constant  Value=0
  Constant2 : Constant  Value=13200
  Constant3 : Constant  Value=0.1
  Constant4 : Constant  Value=5/5*150
  Constant5 : Constant  Value=0.5*2
  Divide : Product  Inputs=*/
  Divide2 : Product  Inputs=*/
  Gain1 : Gain  Gain=sqrt(2/3)
  Gain2 : Gain  Gain=sqrt(2)
  Gain3 : Gain  Gain=sqrt(2)
  Logical Operator1 : Logic  Inputs=3  AllPortsSameDT=off  OutDataTypeStr=boolean
  Logical Operator2 : Logic  Operator=NOT  AllPortsSameDT=off  OutDataTypeStr=boolean
  Logical Operator4 : Logic  Operator=OR  AllPortsSameDT=off  OutDataTypeStr=boolean
  R25 - Sync Check v0.1 : Subsystem  mask(Relay synch check){Ts=Ts}
      mask prompts: Ts "Sampling Time [Sec]"
      mask help:
      | This block checks if the the specified conditions for breaker reclosing
      | are met at both terminals of the circuit breaker. This synch check is
      | intended for use in bus-ties, and service lines.
      |
      | The input bus with the relay parameters should be ordered as follows:
      | 1) VRMSLL
      | 2) IOC
      | 3) TOC
      | 4) dV_threshold
      | 5) angle_threshold
      | 6) dF_threshold
  RMS_Calculator1 : Subsystem  mask{Ts=Ts}
      mask prompts: Ts "Sample Time [Sec]"
  RMS_Calculator2 : Subsystem  mask{Ts=Ts}
      mask prompts: Ts "Sample Time [Sec]"
  S-R Flip-Flop2 : simulink_extras/Flip Flops/S-R Flip-Flop  initial_condition=0
  Scope : Scope  NumInputPorts=3
  Scope2 : Scope  NumInputPorts=2
  Terminator : Terminator
  Terminator1 : Terminator
  Terminator10 : Terminator
  Meas : Outport
  BreakerClose : Outport  Port=2
  wires:
  [Vrms_bus] -> Bus Creator/4  "Vrms_bus"
  [Vrms_line] -> Bus Creator/3  "Vrms_line"
  [PLL_data] -> Bus Creator/5  "PLL_data"
  Gain3/1 -> [Vrms_bus]
  Gain2/1 -> [Vrms_line]
  Divide2/1 -> [Vabc_bus]
  Divide/1 -> [Vabc_line]
  Bus Selector2/1 -> Gain1/1  "<VRMSLL>"
  [RELAY_PARAM] -> Bus Selector2/1
  Gain1/1 -> Divide/2, Divide2/2
  Bus Creator1/1 -> [RELAY_PARAM]
  Constant5/1 -> Bus Creator1/4  "dF_threshold"
  Constant4/1 -> Bus Creator1/3  "angle_threshold"
  Constant2/1 -> Bus Creator1/1  "VRMSLL"
  Constant3/1 -> Bus Creator1/2  "dV_threshold"
  Bus Creator/1 -> Meas/1
  [ReqOpen] -> Logical Operator4/2
  Bus Selector/2 -> [ReqClose]  "<diesel connect>"
  Bus Selector/1 -> [ReqOpen]  "<diesel discon>"
  Constant/1 -> [fault_flag]
  [R25] -> Logical Operator1/3
  S-R Flip-Flop2/2 -> Terminator1/1
  [fault_flag] -> Logical Operator4/1
  Logical Operator2/1 -> Logical Operator1/1
  [fault_flag] -> Logical Operator2/1
  Logical Operator4/1 -> Scope/2, S-R Flip-Flop2/2
  RMS_Calculator1/1(RMS) -> Gain2/1
  RMS_Calculator2/1(RMS) -> Gain3/1
  [Vabc_bus] -> RMS_Calculator2/1(s)
  [Vabc_line] -> RMS_Calculator1/1(s)
  I/1 -> [Iabc]
  V_bus/1 -> Divide2/1
  [RELAY_PARAM] -> R25 - Sync Check v0.1/4(relay_param)
  [Vrms_bus] -> R25 - Sync Check v0.1/1(VPKLN_bus)
  [Vrms_line] -> R25 - Sync Check v0.1/2(VPKLN_line)
  [PLL_data] -> R25 - Sync Check v0.1/3(pll_data)
  R25 - Sync Check v0.1/1(dMeas) -> Bus Creator/1  "R25_Meas"
  [Vabc_line] -> CS Modified PLL1/1(Vabc(pu))
  CS Modified PLL1/2(wt) -> Bus Creator3/2  "wt_line"
  CS Modified PLL/2(wt) -> Bus Creator3/4  "wt_bus"
  [Vabc_bus] -> CS Modified PLL/1(Vabc(pu))
  CS Modified PLL/3(Sin_Cos) -> Terminator/1
  CS Modified PLL/1(Freq) -> Bus Creator3/3  "freq_bus"
  CS Modified PLL1/1(Freq) -> Bus Creator3/1  "freq_line"
  CS Modified PLL1/3(Sin_Cos) -> Terminator10/1
  Bus Creator3/1 -> [PLL_data]
  V_line/1 -> Divide/1
  [ReqClose] -> Scope2/2, Logical Operator1/2
  R25 - Sync Check v0.1/2(R25) -> Scope2/1, [R25], Bus Creator/2  "R25_SyncOK"
  Logical Operator1/1 -> Scope/1, S-R Flip-Flop2/1
  S-R Flip-Flop2/1 -> Bus Creator/6, Scope/3, BreakerClose/1  "Closed"
  [MGCC_cmd] -> Bus Selector/1

== system Auto_microgrid_forecasting_020822/MODEL STABILIZER ==
  Control : Inport
  AllStringInverters : Subsystem
  PV_Array : Subsystem  Commented=on  BlockChoice=FS_Array
      settings: AttributesFormatString=%<BlockChoice>  MemberBlocks=FS_Array,No_Array
      settings: TemplateBlock=|
      | libFSArray/Configurable
      | Subsystem
  Transformer  750kW 13.2-kV/600-V : powerlib/Elements/Three-Phase Transformer (Two Windings)  Winding1Connection=Delta (D1)  Winding2Connection=Yg  CoreType=Three single-phase transformers  SetSaturation=off  Hysteresis=off  DataFile='hysteresis'  SetInitialFlux=off  Measurements=None  UNITS=pu  NominalPower=[ 0.5e6 , 60 ]  Winding1=[13.2e+3 0.003 0.03]  Winding2=[600 0.003 0.03]  Rm=500.02  Lm=inf  L0=0.5  Saturation=[0 0;0.0024 1.2;1 1.52]  InitialFluxes=[ 0.8 , -0.8 , 0.7 ]  BreakLoop=off  DiscreteSolver=Trapezoidal iterative  DataType=off  TransfoNumber=1
  A : PMIOPort  Side=Left
  B : PMIOPort  Port=2  Side=Left
  C : PMIOPort  Port=3  Side=Left
  wires:
  Control/1 -> AllStringInverters/1(Control)
  connections:
  Transformer  750kW 13.2-kV/600-V/RConn2 -- AllStringInverters/LConn2
  Transformer  750kW 13.2-kV/600-V/RConn3 -- AllStringInverters/LConn3
  Transformer  750kW 13.2-kV/600-V/LConn3 -- C/RConn1
  Transformer  750kW 13.2-kV/600-V/RConn1 -- AllStringInverters/LConn1
  Transformer  750kW 13.2-kV/600-V/LConn2 -- B/RConn1
  Transformer  750kW 13.2-kV/600-V/LConn1 -- A/RConn1

== system Auto_microgrid_forecasting_020822/Microgrid controller ==
  note: Figure out how to use f_ref, v_ref
  ProtRelayMeas : Inport
  Bus Creator : BusCreator  Inputs=6
  Bus Selector : BusSelector  OutputSignals=BESS PQ cmd,resync,f setpoint,V setpoint,BESS mode,BESS switch
  Demux1 : Demux  Outputs=2
  ResyncControl : Subsystem
  BESS_Control : Outport
  wires:
  Bus Creator/1 -> BESS_Control/1
  Demux1/2 -> Bus Creator/2  "q_ref"
  Demux1/1 -> Bus Creator/1  "p_ref"
  ProtRelayMeas/1 -> ResyncControl/1(ProtRelayMeas)
  ResyncControl/1(f_ref) -> Bus Creator/3  "f_ref"
  ResyncControl/2(v_ref) -> Bus Creator/4  "v_ref"
  [MGCC_cmd] -> Bus Selector/1
  Bus Selector/1 -> Demux1/1  "<BESS PQ cmd>"
  Bus Selector/2 -> ResyncControl/4(<StartResync>)  "<resync>"
  Bus Selector/5 -> Bus Creator/5  "<BESS mode>"
  Bus Selector/6 -> Bus Creator/6  "<BESS switch>"
  Bus Selector/3 -> ResyncControl/2(f setpoint)  "<f setpoint>"
  Bus Selector/4 -> ResyncControl/3(V setpoint)  "<V setpoint>"

== system Auto_microgrid_forecasting_020822/Resource Timeseries ==
  note: Load Time Series
  note: Resource Time Series
  1-D Lookup Table : Lookup_n-D  NumberOfTableDimensions=1  BreakpointsForDimension1=ts.TimeElapsed  Table=ts.Cup_WS_38m  InternalRulePriority=Speed  RndMeth=Simplest  InputSameDT=on
  1-D Lookup Table1 : Lookup_n-D  NumberOfTableDimensions=1  BreakpointsForDimension1=ts.TimeElapsed  Table=ts.Solar  InternalRulePriority=Speed  RndMeth=Simplest  InputSameDT=on
  1-D Lookup Table2 : Lookup_n-D  NumberOfTableDimensions=1  BreakpointsForDimension1=ts.TimeElapsed  Table=ts.Sonic_Temp_41  InternalRulePriority=Speed  RndMeth=Simplest  InputSameDT=on
  1-D Lookup Table3 : Lookup_n-D  NumberOfTableDimensions=1  BreakpointsForDimension1=pq_ts.Time  Table=pq_ts.Data.actPower  InternalRulePriority=Speed  RndMeth=Simplest  InputSameDT=on
  1-D Lookup Table4 : Lookup_n-D  NumberOfTableDimensions=1  BreakpointsForDimension1=pq_ts.Time  Table=pq_ts.Data.recPower  InternalRulePriority=Speed  RndMeth=Simplest  InputSameDT=on
  Clock : Clock
  tag scope: SR_ts_wm2=global, Temp_ts=global, VARP=global, VARQ=global, WS_ts=global
  wires:
  1-D Lookup Table/1 -> [WS_ts]
  1-D Lookup Table2/1 -> [Temp_ts]
  1-D Lookup Table1/1 -> [SR_ts_wm2]
  1-D Lookup Table3/1 -> [VARP]
  Clock/1 -> 1-D Lookup Table3/1, 1-D Lookup Table1/1, 1-D Lookup Table4/1, 1-D Lookup Table2/1, 1-D Lookup Table/1
  1-D Lookup Table4/1 -> [VARQ]

== system Auto_microgrid_forecasting_020822/Stab1 ==
  Control : Inport
  AllStringInverters : Subsystem
  Transformer  750kW 13.2-kV/600-V : powerlib/Elements/Three-Phase Transformer (Two Windings)  Winding1Connection=Delta (D1)  Winding2Connection=Yg  CoreType=Three single-phase transformers  SetSaturation=off  Hysteresis=off  DataFile='hysteresis'  SetInitialFlux=off  Measurements=None  UNITS=pu  NominalPower=[ 0.5e6 , 60 ]  Winding1=[13.2e+3 0.003 0.03]  Winding2=[600 0.003 0.03]  Rm=500.02  Lm=inf  L0=0.5  Saturation=[0 0;0.0024 1.2;1 1.52]  InitialFluxes=[ 0.8 , -0.8 , 0.7 ]  BreakLoop=off  DiscreteSolver=Trapezoidal iterative  DataType=off  TransfoNumber=1
  A : PMIOPort  Side=Left
  B : PMIOPort  Port=2  Side=Left
  C : PMIOPort  Port=3  Side=Left
  wires:
  Control/1 -> AllStringInverters/1(Control)
  connections:
  Transformer  750kW 13.2-kV/600-V/RConn2 -- AllStringInverters/LConn2
  Transformer  750kW 13.2-kV/600-V/RConn1 -- AllStringInverters/LConn1
  Transformer  750kW 13.2-kV/600-V/LConn1 -- A/RConn1
  Transformer  750kW 13.2-kV/600-V/RConn3 -- AllStringInverters/LConn3
  Transformer  750kW 13.2-kV/600-V/LConn3 -- C/RConn1
  Transformer  750kW 13.2-kV/600-V/LConn2 -- B/RConn1
